simulink model "SM_OPAMPs"  (R2023b)
settings: Solver=VariableStepAuto  StartTime=0.0  StopTime=5  RelTol=1e-3
values from neighbouring files (symbols this model uses):
  C1 = 100e-9    (= 1e-07)    [Opamp.m]    (also in ResCap.mat)
  C2 = C1    (= 1e-07)    [Opamp.m]    (also in ResCap.mat)
  R1 = 5e+6    (= 5000000)    [Opamp.m]    (also in ResCap.mat)
  R2 = R1    (= 5000000)    [Opamp.m]    (also in ResCap.mat)
  R3 = R2    (= 5000000)    [Opamp.m]    (also in ResCap.mat)

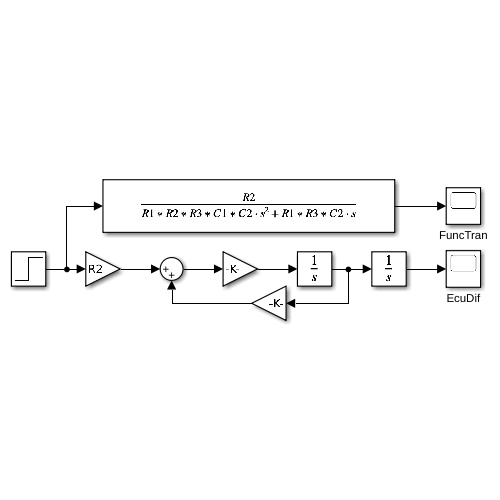
[thumbnail: Simulink's stored preview of the top-level diagram]
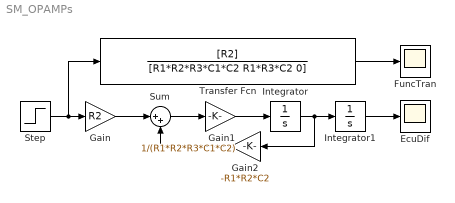
== system SM_OPAMPs ==
  EcuDif : Scope
  FuncTran : Scope
  Gain : Gain  Gain=R2
  Gain1 : Gain  Gain=1/(R1*R2*R3*C1*C2)
  Gain2 : Gain  Gain=-R1*R2*C2
  Integrator : Integrator
  Integrator1 : Integrator
  Step : Step  Time=0  After=5  SampleTime=0
  Sum : Sum  Inputs=|++
  Transfer Fcn : TransferFcn  Numerator=[R2]  Denominator=[R1*R2*R3*C1*C2 R1*R3*C2 0]
  wires:
  Integrator1/1 -> EcuDif/1
  Step/1 -> Transfer Fcn/1, Gain/1
  Gain2/1 -> Sum/2
  Integrator/1 -> Integrator1/1, Gain2/1
  Sum/1 -> Gain1/1
  Gain1/1 -> Integrator/1
  Gain/1 -> Sum/1
  Transfer Fcn/1 -> FuncTran/1
